simulink model "pen_linear_close"  (R2018a)
settings: Solver=VariableStepAuto  StartTime=0.0  StopTime=10.0  RelTol=1e-3
undefined symbols (not defined in the file): A, B, C, K, ts
settings Model: Creator=ros  LastModifiedBy=ros

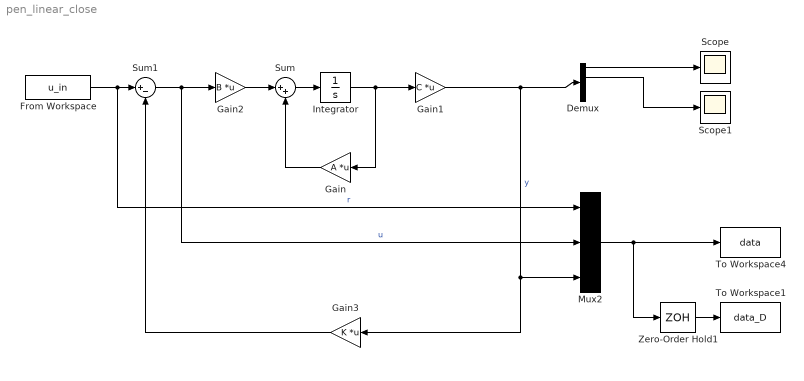
== system pen_linear_close ==
  Demux : Demux
  From Workspace : FromWorkspace  VariableName=u_in  SampleTime=0.001
  Gain : Gain  Gain=A  Multiplication=Matrix(K*u)
  Gain1 : Gain  Gain=C  Multiplication=Matrix(K*u)
  Gain2 : Gain  Gain=B  Multiplication=Matrix(K*u)
  Gain3 : Gain  Gain=K  Multiplication=Matrix(K*u)
  Integrator : Integrator  InitialCondition=[0,0.5,0,0]
  Mux2 : Mux  Inputs=3
      settings: DisplayOption=signals
  Scope : Scope
  Scope1 : Scope
  Sum : Sum  Inputs=|++
  Sum1 : Sum  Inputs=|+-
  To Workspace1 : ToWorkspace  VariableName=data_D  SaveFormat=Timeseries  SampleTime=-1
  To Workspace4 : ToWorkspace  VariableName=data  SaveFormat=Timeseries  SampleTime=-1
  Zero-Order Hold1 : ZeroOrderHold  SampleTime=ts
  wires:
  Integrator/1 -> Gain1/1, Gain/1
  Gain/1 -> Sum/2
  Gain2/1 -> Sum/1
  Sum/1 -> Integrator/1
  Gain1/1 -> Gain3/1, Mux2/3, Demux/1  "y"
  Mux2/1 -> Zero-Order Hold1/1, To Workspace4/1
  Zero-Order Hold1/1 -> To Workspace1/1
  Gain3/1 -> Sum1/2
  Sum1/1 -> Mux2/2, Gain2/1  "u"
  From Workspace/1 -> Mux2/1, Sum1/1  "r"
  Demux/1 -> Scope/1
  Demux/2 -> Scope1/1
